simulink library "LookupLib"  (R2020a)
settings: Solver=VariableStepAuto  StartTime=0.0  StopTime=10.0  RelTol=1e-3
settings Model: Creator=harjo  LastModifiedBy=harjo

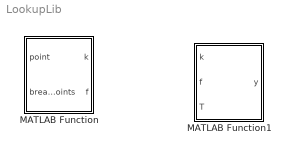
== system LookupLib ==
  MATLAB Function : MATLAB Function  TreatAsAtomicUnit=on
  MATLAB Function1 : MATLAB Function  TreatAsAtomicUnit=on

== matlab function LookupLib/MATLAB Function1 ==
  data: k input; y output; f input; T input
function y = fcn(k,f,T)
if(f == 0)
    y = T(k);
else
    diff = T(k+1) - T(k);
    y = T(k) + f*diff;
end

== matlab function LookupLib/MATLAB Function ==
  data: point input; k output; breakPoints input; f output
function [k,f] = fcn(point,breakPoints)
if(point >= breakPoints)
    k = length(breakPoints);
    f = 0;
    return
elseif(point <= breakPoints)
    k = 1;
    f = 0;
else
    endIndex = length(breakPoints);
    for i = 1:length(breakPoints)
        if(point <= breakPoints(i))
            endIndex = i;
        break
        end
    end
    k = endIndex - 1;
    f = (point - breakPoints(k))/(breakPoints(endIndex) - breakPoints(k));
end
